simulink model "P4"  (R2015b)
settings: Solver=VariableStepAuto  StartTime=0.0  StopTime=10  RelTol=1e-3
libraries: fl_lib x19, nesl_utility x3
settings Model: Creator=xmax1946  LastModifiedBy=xmax1946

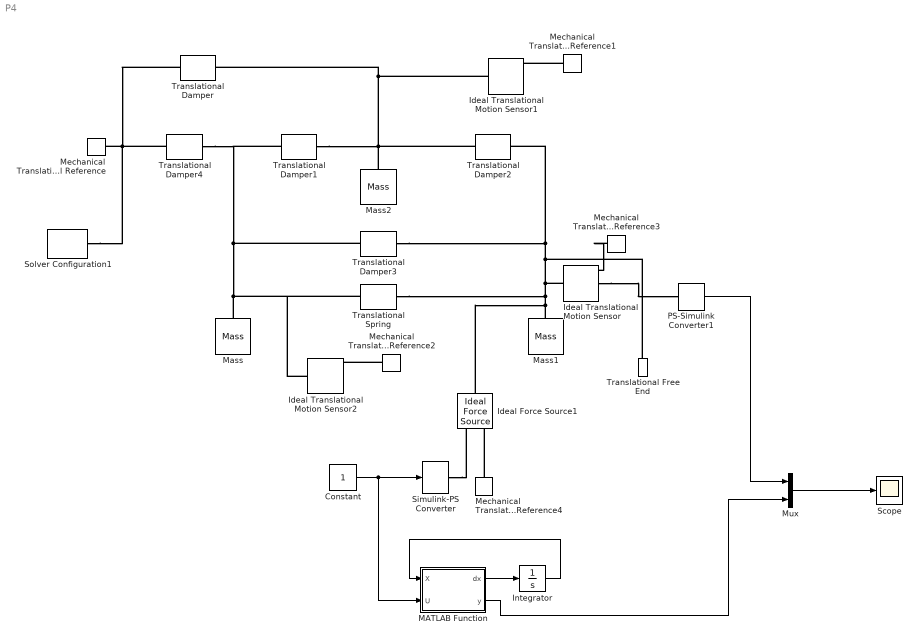
== system P4 ==
  Constant : Constant
  Ideal Force Source1 : fl_lib/Mechanical/Mechanical Sources/Ideal Force Source
  Ideal Translational Motion Sensor : fl_lib/Mechanical/Mechanical Sensors/Ideal Translational Motion Sensor  offset=0 m
  Ideal Translational Motion Sensor1 : fl_lib/Mechanical/Mechanical Sensors/Ideal Translational Motion Sensor  offset=0 m
  Ideal Translational Motion Sensor2 : fl_lib/Mechanical/Mechanical Sensors/Ideal Translational Motion Sensor  offset=0 m
  Integrator : Integrator  InitialCondition=[0;0;0;0;0;0]
  MATLAB Function : MATLAB Function  TreatAsAtomicUnit=on
  Mass : fl_lib/Mechanical/Translational Elements/Mass  mass=2 kg  v_specify=off  v_priority=None  v=0 m/s  f_specify=off  f_priority=None  f=0 N
  Mass1 : fl_lib/Mechanical/Translational Elements/Mass  mass=1 kg  v_specify=off  v_priority=None  v=0 m/s  f_specify=off  f_priority=None  f=0 N
  Mass2 : fl_lib/Mechanical/Translational Elements/Mass  mass=1 kg  v_specify=off  v_priority=None  v=0 m/s  f_specify=off  f_priority=None  f=0 N
  Mechanical Translational Reference{,1..4} (5 alike) : fl_lib/Mechanical/Translational Elements/Mechanical Translational Reference
  Mux : Mux  Inputs=2
  PS-Simulink Converter1 : nesl_utility/PS-Simulink Converter  PhysicalDomain=network_engine_domain  SubClassName=ps_output  LeftPortType=input  RightPortType=output  PseudoPeriodic=off  Frequencies=[]  Unit=1  AffineConversion=off
  Scope : Scope
  Simulink-PS Converter : nesl_utility/Simulink-PS Converter  PhysicalDomain=network_engine_domain  SubClassName=ps_input  LeftPortType=input  RightPortType=output  PseudoPeriodic=off  Frequencies=[]  NoiseDistribution=none  NoiseParameters=[]  Unit=1  AffineConversion=off  InputFiltering=off  SimscapeFilterOrder=1  InputFilterTimeConstant=0.001  UdotUserProvided=1
  Solver Configuration1 : nesl_utility/Solver Configuration  PhysicalDomain=network_engine_domain  SubClassName=solver  LeftPortType=input  RightPortType=generic  Accelerate=off  Tones=[]  Harmonics=[]  SimulateNoise=off  Profile=off  UseLocalSampling=off  EnableSwitchedLinearOptims=on  FrequencyDomain=off  UseCCode=off  RelTol=0.001  AbsTol=1e-06  MinStep=1e-09  ToWorkspace=off  RevertToSquareIcSolve=off  NumHomotopyIterations=100  PhasorMode=off  PhasorModeNumHarmonics=1  DoDC=off  ResidualTolerance=1e-09  UseLocalSolver=off  LocalSolverChoice=NE_BACKWARD_EULER_ADVANCER  LocalSolverSampleTime=0.001  DoFixedCost=off  MaxNonlinIter=3  MaxModeIter=2  LinearAlgebra=Sparse  DelaysMemoryBudget=1024  AutomaticFiltering=on  FilteringTimeConstant=0.001
  Translational Damper{,1..4} (5 alike) : fl_lib/Mechanical/Translational Elements/Translational Damper  D=1 N/(m/s)  v_specify=off  v_priority=None  v=0 m/s  f_specify=off  f_priority=None  f=0 N
  Translational Free End : fl_lib/Mechanical/Translational Elements/Translational Free End  v_specify=off  v_priority=None  v=0 m/s
  Translational Spring : fl_lib/Mechanical/Translational Elements/Translational Spring  spr_rate=2 N/m  v_specify=off  v_priority=None  v=0 m/s  f_specify=off  f_priority=None  f=0 N  x_specify=off  x_priority=None  x=0 m
  wires:
  Constant/1 -> MATLAB Function/2(U), Simulink-PS Converter/1
  MATLAB Function/1(dx) -> Integrator/1
  MATLAB Function/2(y) -> Mux/2
  PS-Simulink Converter1/1 -> Mux/1
  Mux/1 -> Scope/1
  Integrator/1 -> MATLAB Function/1(X)
  connections:
  Translational Damper4/LConn1 -- Translational Damper/LConn1 -- Mechanical Translational Reference/LConn1 -- Solver Configuration1/RConn1
  Mass/LConn1 -- Translational Damper4/RConn1 -- Translational Damper1/LConn1 -- Translational Damper3/LConn1 -- Ideal Translational Motion Sensor2/LConn1 -- Translational Spring/LConn1
  Mass2/LConn1 -- Translational Damper2/LConn1 -- Translational Damper1/RConn1 -- Ideal Translational Motion Sensor1/LConn1 -- Translational Damper/RConn1
  Mass1/LConn1 -- Ideal Force Source1/LConn1 -- Translational Spring/RConn1 -- Ideal Translational Motion Sensor/LConn1 -- Translational Damper2/RConn1 -- Translational Damper3/RConn1 -- Translational Free End/LConn1
  Mechanical Translational Reference4/LConn1 -- Ideal Force Source1/RConn2
  Simulink-PS Converter/RConn1 -- Ideal Force Source1/RConn1
  Mechanical Translational Reference3/LConn1 -- Ideal Translational Motion Sensor/RConn1
  Mechanical Translational Reference1/LConn1 -- Ideal Translational Motion Sensor1/RConn1
  Mechanical Translational Reference2/LConn1 -- Ideal Translational Motion Sensor2/RConn1
  Ideal Translational Motion Sensor/RConn2 -- PS-Simulink Converter1/LConn1

== matlab function P4/MATLAB Function ==
  data: dx output; X input; y output; U input
function [dx,y] = fs(X,U)
m1=2;
m2=1;
m3=1;
v1=1;
v2=1;
v3=1;
v4=1;
v5=1;
k=2;
A=[0,1,0,0,0,0;
  -k/m1,(-v2-v4-v1)/m1,k/m1,v2/m1,0,v4/m1
  0,0,0,1,0,0 
  k/m2,v2/m2,-k/m2,(-v2-v5)/m2,0,v5/m2
  0,0,0,0,0,1
  0,v4/m3,0,v5/m3,0,(-v4-v3-v5)/m3
    ];
B=[0;0;0;1/m2;0;0];
C=[0,0,0,1,0,0];
u=U;
dx=A*X+B*u;
y=C*X;
